simulink model "PID_FF_Motor_con_carga"  (R2018a)
settings: Solver=VariableStepAuto  StartTime=0.0  StopTime=inf  RelTol=1e-6
libraries: simulink x3
settings Model: PauseTimes=1  Creator=antonio  LastModifiedBy=roiro
settings CodeAppCC: StateflowObjectComments=on

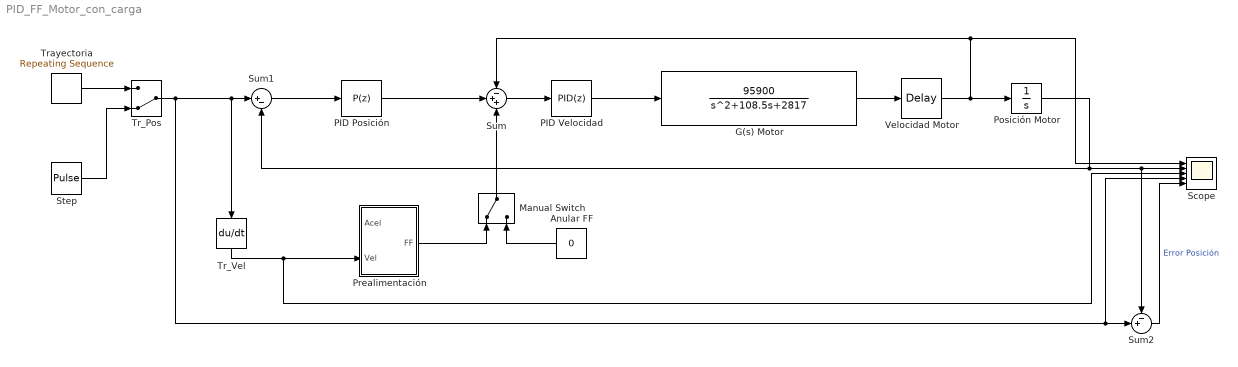
== system PID_FF_Motor_con_carga ==
  Anular FF : Constant  Value=0
  G(s) Motor : TransferFcn  Numerator=[95900]  Denominator=[1 108.5 2817]
  Manual Switch : ManualSwitch
  PID Posición : simulink/Continuous/PID Controller  Controller=P  TimeDomain=Discrete-time  SampleTime=0.005  IntegratorMethod=Forward Euler  FilterMethod=Forward Euler  Form=Parallel  UseFilter=on  ControllerParametersSource=internal  P=5.9475806451613  I=0  D=0  N=100  InitialConditionSource=internal  InitialConditionForIntegrator=0  InitialConditionForFilter=0  ExternalReset=none  LimitOutput=off  UpperSaturationLimit=8  LowerSaturationLimit=-8  LinearizeAsGain=on  AntiWindupMode=back-calculation  Kb=0  TrackingMode=off  Kt=1  PParamMin=[]  PParamMax=[]  IParamMin=[]  IParamMax=[]  DParamMin=[]  DParamMax=[]  NParamMin=[]  NParamMax=[]  KbParamMin=[]  KbParamMax=[]  KtParamMin=[]  KtParamMax=[]  POutMin=[]  POutMax=[]  IOutMin=[]  IOutMax=[]  DOutMin=[]  DOutMax=[]  NOutMin=[]  NOutMax=[]  KbOutMin=[]  KbOutMax=[]  KtOutMin=[]  KtOutMax=[]  IntegratorOutMin=[]  IntegratorOutMax=[]  FilterOutMin=[]  FilterOutMax=[]  SumOutMin=[]  SumOutMax=[]  SumI1OutMin=[]  SumI1OutMax=[]  SumI2OutMin=[]  SumI2OutMax=[]  SumI3OutMin=[]  SumI3OutMax=[]  SumDOutMin=[]  SumDOutMax=[]  SaturationOutMin=[]  SaturationOutMax=[]  IntegratorContinuousStateAttributes=''  IntegratorStateMustResolveToSignalObject=off  IntegratorRTWStateStorageClass=Auto  FilterContinuousStateAttributes=''  FilterStateMustResolveToSignalObject=off  FilterRTWStateStorageClass=Auto  DifferentiatorICPrevScaledInput=0  DifferentiatorOutMin=[]  DifferentiatorOutMax=[]  FilterDiffOutCoefMin=[]  FilterDiffOutCoefMax=[]  SumDenOutMin=[]  SumDenOutMax=[]  SumNumOutMin=[]  SumNumOutMax=[]  ReciprocalOutMin=[]  ReciprocalOutMax=[]  DivideOutMin=[]  DivideOutMax=[]  TunerSelectOption=Transfer Function Based (PID Tuner App)
  PID Velocidad : simulink/Continuous/PID Controller  Controller=PID  TimeDomain=Discrete-time  SampleTime=0.005  IntegratorMethod=Forward Euler  FilterMethod=Forward Euler  Form=Parallel  UseFilter=on  ControllerParametersSource=internal  P=0.0413671895295389  I=1.08422696420092  D=0.000106482449648477  N=72.5163299758294  InitialConditionSource=internal  InitialConditionForIntegrator=0  InitialConditionForFilter=0  ExternalReset=none  LimitOutput=on  UpperSaturationLimit=255  LowerSaturationLimit=-255  LinearizeAsGain=on  AntiWindupMode=back-calculation  Kb=8  TrackingMode=off  Kt=1  PParamMin=[]  PParamMax=[]  IParamMin=[]  IParamMax=[]  DParamMin=[]  DParamMax=[]  NParamMin=[]  NParamMax=[]  KbParamMin=[]  KbParamMax=[]  KtParamMin=[]  KtParamMax=[]  POutMin=[]  POutMax=[]  IOutMin=[]  IOutMax=[]  DOutMin=[]  DOutMax=[]  NOutMin=[]  NOutMax=[]  KbOutMin=[]  KbOutMax=[]  KtOutMin=[]  KtOutMax=[]  IntegratorOutMin=[]  IntegratorOutMax=[]  FilterOutMin=[]  FilterOutMax=[]  SumOutMin=[]  SumOutMax=[]  SumI1OutMin=[]  SumI1OutMax=[]  SumI2OutMin=[]  SumI2OutMax=[]  SumI3OutMin=[]  SumI3OutMax=[]  SumDOutMin=[]  SumDOutMax=[]  SaturationOutMin=[]  SaturationOutMax=[]  IntegratorContinuousStateAttributes=''  IntegratorStateMustResolveToSignalObject=off  IntegratorRTWStateStorageClass=Auto  FilterContinuousStateAttributes=''  FilterStateMustResolveToSignalObject=off  FilterRTWStateStorageClass=Auto  DifferentiatorICPrevScaledInput=0  DifferentiatorOutMin=[]  DifferentiatorOutMax=[]  FilterDiffOutCoefMin=[]  FilterDiffOutCoefMax=[]  SumDenOutMin=[]  SumDenOutMax=[]  SumNumOutMin=[]  SumNumOutMax=[]  ReciprocalOutMin=[]  ReciprocalOutMax=[]  DivideOutMin=[]  DivideOutMax=[]  TunerSelectOption=Transfer Function Based (PID Tuner App)
  Posición Motor : Integrator
  Prealimentación : Subsystem
  Scope : Scope  NumInputPorts=5
  Step : DiscretePulseGenerator  PulseType=Time based  Amplitude=5000  Period=4  PulseWidth=50
  Sum : Sum  Inputs=-++
  Sum1 : Sum  Inputs=|+-
  Sum2 : Sum  Inputs=-+|
  Tr_Pos : ManualSwitch  CurrentSetting=0
  Tr_Vel : Derivative
  "Trayectoria " : simulink/Sources/Repeating Sequence  rep_seq_t=Time  rep_seq_y=Tr
  Velocidad Motor : TransportDelay  DelayTime=0.00662
  wires:
  Anular FF/1 -> Manual Switch/2
  Sum1/1 -> PID Posición/1
  Prealimentación/1(FF) -> Manual Switch/1
  Velocidad Motor/1 -> Sum/1, Scope/1, Posición Motor/1
  Sum/1 -> PID Velocidad/1
  PID Velocidad/1 -> G(s) Motor/1
  PID Posición/1 -> Sum/2
  G(s) Motor/1 -> Velocidad Motor/1
  Tr_Pos/1 -> Scope/4, Sum2/2, Sum1/1, Tr_Vel/1
  Tr_Vel/1 -> Scope/3, Prealimentación/2(Vel)
  Manual Switch/1 -> Sum/3
  "Trayectoria "/1 -> Tr_Pos/1
  Step/1 -> Tr_Pos/2
  Sum2/1 -> Scope/5  "Error Posición"
  Posición Motor/1 -> Sum2/1, Scope/2, Sum1/2

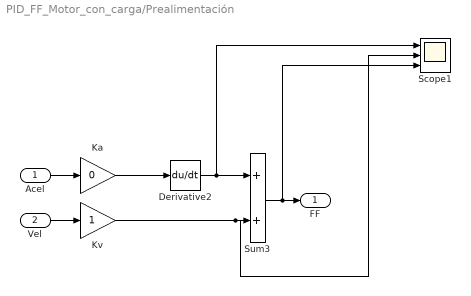
== system PID_FF_Motor_con_carga/Prealimentación ==
  Acel : Inport
  Vel : Inport  Port=2
  Derivative2 : Derivative
  Ka : Gain  Gain=0
  Kv : Gain
  Scope1 : Scope  NumInputPorts=3
  Sum3 : Sum
  FF : Outport
  wires:
  Vel/1 -> Kv/1
  Acel/1 -> Ka/1
  Ka/1 -> Derivative2/1
  Derivative2/1 -> Scope1/1, Sum3/1
  Sum3/1 -> Scope1/3, FF/1
  Kv/1 -> Scope1/2, Sum3/2
